simulink model "Dijkstra_Optimization_2"  (R2015b)
settings: Solver=FixedStepDiscrete  SolverMode=SingleTasking  StartTime=0.0  StopTime=10e-5  RelTol=1e-3
libraries: shlslibv1 x995
(part 6 of 6)

== system Dijkstra_Optimization_2/Dijkstra/Subsystem9/Subsystem10/min_distance ==
  In1 : Inport
  In2 : Inport  Port=2
  In3 : Inport  Port=3
  In4 : Inport  Port=4
  In5 : Inport  Port=5
  In6 : Inport  Port=6
  In7 : Inport  Port=7
  In8 : Inport  Port=8
  Add1 : shlslibv1/Math Functions/Add  syn_add_opr=++  syn_out_f=Full Precision  syn_out_wl=16  syn_out_fl=8  syn_out_dt=signed  syn_out_sat=off  syn_out_rnd=Floor (Truncate)  synBlockType=primitive  synLatency=0  synBlockId=96  syn_sum_of_rows=off  syn_inh_port=off  syn_inh_st=on  syn_inh_stf=1  syn_en_pipe=off  syn_pipe_stg=syn_max_pipeline  syn_flow_ctrl=off
  Binary Logic1 : shlslibv1/Math Functions/Binary Logic  syn_binlog_exp=a&b&c&d  synBlockType=primitive  synLatency=0  synBlockId=13
  Convert1 : shlslibv1/Signal Operations/Convert  syn_preshift_opr=none  syn_preshift_bits=0  syn_preshift_val=0  syn_out_f=Specify  syn_out_wl=50  syn_out_fl=0  syn_out_dt_sync=unsigned  syn_out_sat=off  syn_out_rnd=Floor (Truncate)  syn_inh_port=off  syn_inh_st=off  syn_inh_stf=1  syn_en_pipe=off  syn_pipe_stg=syn_max_pipeline  syn_flow_ctrl=off  syn_sat_op=off  synBlockType=primitive  synLatency=0  synBlockId=4
  Convert3 : shlslibv1/Signal Operations/Convert  syn_preshift_opr=none  syn_preshift_bits=0  syn_preshift_val=0  syn_out_f=Specify  syn_out_wl=50  syn_out_fl=0  syn_out_dt_sync=unsigned  syn_out_sat=off  syn_out_rnd=Floor (Truncate)  syn_inh_port=off  syn_inh_st=off  syn_inh_stf=1  syn_en_pipe=off  syn_pipe_stg=syn_max_pipeline  syn_flow_ctrl=off  syn_sat_op=off  synBlockType=primitive  synLatency=0  synBlockId=4
  Mux2 : shlslibv1/Signal Operations/Mux  syn_in_nb=4  syn_out_f=Full Precision  syn_out_wl=11  syn_out_fl=52  syn_out_dt=unsigned  syn_en_se=off  synBlockType=primitive  synLatency=0  synBlockId=16
  "dist[u]  INT_MAX " : shlslibv1/Math Functions/Comparator  syn_comp_opr=a!=b  syn_comp_const=on  syn_comp_val=64  syn_en_se=off  synBlockType=primitive  synLatency=0  synBlockId=14
  dist[u][u][v]  dist[v] : shlslibv1/Math Functions/Comparator  syn_comp_opr=a<b  syn_comp_const=off  syn_comp_val=64  syn_en_se=off  synBlockType=primitive  synLatency=0  synBlockId=14
  graph[u][v] : shlslibv1/Math Functions/Comparator  syn_comp_opr=a!=b  syn_comp_const=on  syn_comp_val=0  syn_en_se=off  synBlockType=primitive  synLatency=0  synBlockId=14
  "v]\t" : shlslibv1/Math Functions/Comparator  syn_comp_opr=a==b  syn_comp_const=on  syn_comp_val=0  syn_en_se=off  synBlockType=primitive  synLatency=0  synBlockId=14
  Out1 : Outport
  Out2 : Outport  Port=2
  wires:
  In5/1 -> Mux2/2
  In6/1 -> Mux2/3
  dist[u][u][v]  dist[v]/1 -> Binary Logic1/1
  "dist[u]  INT_MAX "/1 -> Binary Logic1/2
  graph[u][v]/1 -> Binary Logic1/3
  Add1/1 -> Convert3/1, dist[u][u][v]  dist[v]/1
  Binary Logic1/1 -> Convert1/1
  "v]\t"/1 -> Binary Logic1/4
  Mux2/1 -> Add1/2, graph[u][v]/1
  In4/1 -> "v]\t"/1
  Convert3/1 -> Out1/1
  Convert1/1 -> Out2/1
  In1/1 -> dist[u][u][v]  dist[v]/2
  In2/1 -> "dist[u]  INT_MAX "/1, Add1/1
  In3/1 -> Mux2/1
  In8/1 -> Mux2/5
  In7/1 -> Mux2/4
